simulink model "Project_5_lin_s_7_5"  (Simulink 8.4)
settings: Solver=ode5  StartTime=0.0  StopTime=10.0  FixedStep=0.01  RelTol=1e-3
values from neighbouring files (symbols this model uses):
  da = da_d*d2r    (= 0)    [Project_5_m.m]
  de = de_d*d2r    (= 0)    [Project_5_m.m]
  dr = dr_d*d2r    (= -0.0349065850399)    [Project_5_m.m]
  r2d = 180/pi    (= 57.2957795131)    [Project_5_m.m]
  xo = [0 0 0 0 0 0 0 0 0]    [Project_5_m.m]
undefined symbols (not defined in the file or in its folder): A, B, C, D
settings Model: Creator=cmc4177  LastModifiedBy=cmc4177
settings DataIOCC: LimitDataPoints=off  SaveOutput=off  SaveTime=off
settings OptimizationCC: ExpressionDepthLimit=128
settings DebuggingCC: UnderspecifiedInitializationDetection=Simplified  MergeDetectMultiDrivingBlocksExec=error  StateNameClashWarn=none

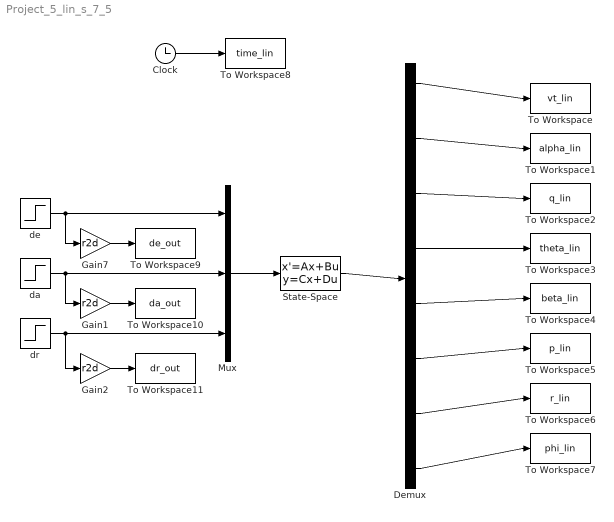
== system Project_5_lin_s_7_5 ==
  Clock : Clock
  Demux : Demux  Outputs=8
  Gain1 : Gain  Gain=r2d
  Gain2 : Gain  Gain=r2d
  Gain7 : Gain  Gain=r2d
  Mux : Mux  Inputs=3
  State-Space : StateSpace  A=A  B=B  C=C  D=D  X0=xo
  To Workspace : ToWorkspace  VariableName=vt_lin  SampleTime=-1
  To Workspace1 : ToWorkspace  VariableName=alpha_lin  SampleTime=-1
  To Workspace10 : ToWorkspace  VariableName=da_out  SampleTime=-1
  To Workspace11 : ToWorkspace  VariableName=dr_out  SampleTime=-1
  To Workspace2 : ToWorkspace  VariableName=q_lin  SampleTime=-1
  To Workspace3 : ToWorkspace  VariableName=theta_lin  SampleTime=-1
  To Workspace4 : ToWorkspace  VariableName=beta_lin  SampleTime=-1
  To Workspace5 : ToWorkspace  VariableName=p_lin  SampleTime=-1
  To Workspace6 : ToWorkspace  VariableName=r_lin  SampleTime=-1
  To Workspace7 : ToWorkspace  VariableName=phi_lin  SampleTime=-1
  To Workspace8 : ToWorkspace  VariableName=time_lin  SampleTime=-1
  To Workspace9 : ToWorkspace  VariableName=de_out  SampleTime=-1
  da : Step  After=da  SampleTime=0
  de : Step  After=de  SampleTime=0
  dr : Step  After=dr  SampleTime=0
  wires:
  de/1 -> Mux/1, Gain7/1
  da/1 -> Mux/2, Gain1/1
  dr/1 -> Mux/3, Gain2/1
  Mux/1 -> State-Space/1
  State-Space/1 -> Demux/1
  Demux/1 -> To Workspace/1
  Demux/2 -> To Workspace1/1
  Demux/3 -> To Workspace2/1
  Demux/4 -> To Workspace3/1
  Demux/5 -> To Workspace4/1
  Demux/6 -> To Workspace5/1
  Demux/7 -> To Workspace6/1
  Demux/8 -> To Workspace7/1
  Clock/1 -> To Workspace8/1
  Gain7/1 -> To Workspace9/1
  Gain1/1 -> To Workspace10/1
  Gain2/1 -> To Workspace11/1
